simulink model "QP_NMPC_FSR"  (R2023a)
settings: Solver=ode4  StartTime=0.0  StopTime=T  RelTol=1e-3
InitFcn:
  | run('NLMPC_QUADCOPTER.m');
values from neighbouring files (symbols this model uses):
  g = 9.81    [NLMPC_QUADCOPTER.m]    (also in NMPC_XFcn.m)
  m = 0.85    [NLMPC_QUADCOPTER.m]    (also in NMPC_XFcn.m)
  PSI = zeros(1, length(PP))    [LOAD_NMPC.m]
undefined symbols (not defined in the file or in its folder): PP
libraries: robotcorelib x1, mpclib x1, uavutilslib x1
settings Model: ModifiedByFormat=salvatoregranata  Creator=salvatoregranata  LastModifiedBy=salvatoregranata

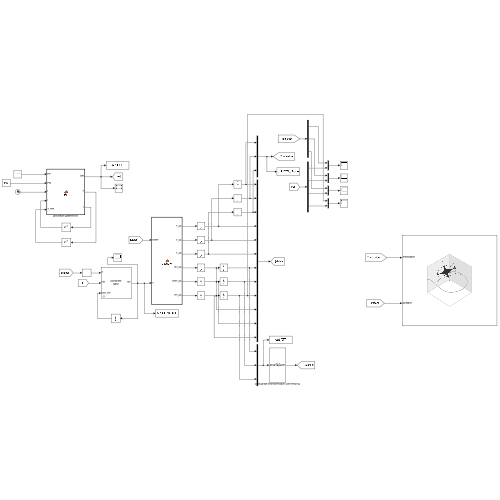
[thumbnail: Simulink's stored preview of the top-level diagram]
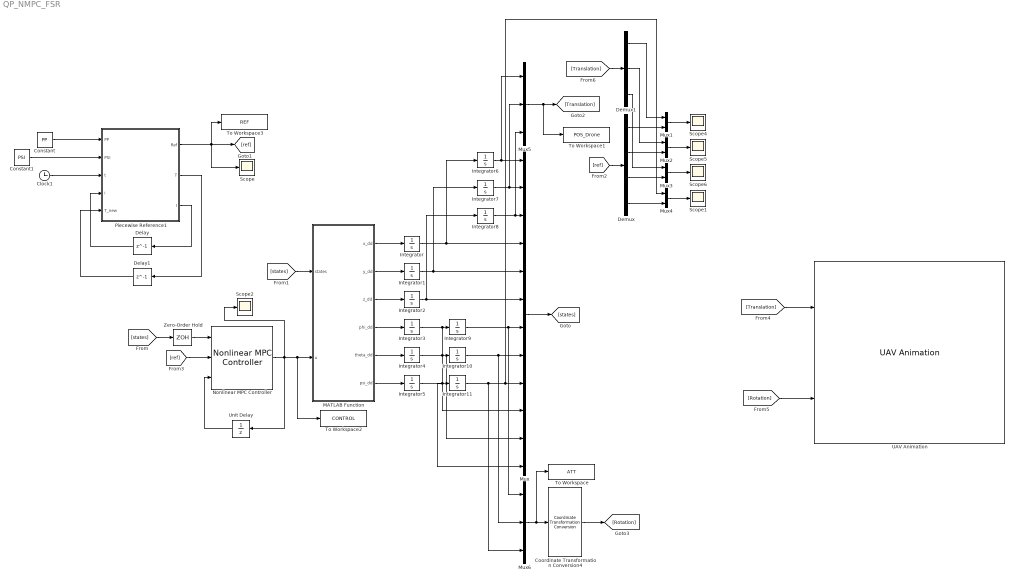
== system QP_NMPC_FSR ==
  Clock1 : Clock
  Constant : Constant  Value=PP
  Constant1 : Constant  Value=PSI
  Coordinate Transformation Conversion4 : robotcorelib/Coordinate Transformation Conversion  InputRepresentation=Euler Angles  InputEulerSequence=XYZ  ShowTrVecInputPort=on  OutputRepresentation=Quaternion  OutputEulerSequence=ZYX  ShowTrVecOutputPort=on  SimulateUsing=Interpreted execution
  Delay : Delay  DelayLength=1  InitialCondition=1  SampleTime=0.001
  Delay1 : Delay  DelayLength=1  SampleTime=0.001
  Demux : Demux
  Demux1 : Demux  Outputs=3
  Integrator{,1..5,9..10} (8 alike) : Integrator
  Integrator11 : Integrator  InitialCondition=PSI(1,1)
  Integrator6 : Integrator  InitialCondition=PP(1,1)
  Integrator7 : Integrator  InitialCondition=PP(2,1)
  Integrator8 : Integrator  InitialCondition=PP(3,1)
  MATLAB Function : MATLAB Function  TreatAsAtomicUnit=on
  Mux : Mux  Inputs=12
  Mux{1..4} (4 alike) : Mux  Inputs=2
  Mux5 : Mux  Inputs=3
  Mux6 : Mux  Inputs=3
  Nonlinear MPC Controller : mpclib/Nonlinear MPC Controller  nlmpcobj=my_NMPC  UseObjectTs=on  UseMEX=off  md_enabled=off  mvtarget_enabled=off  param_enabled=off  cost_enabled=off  mvseq_enabled=off  stateseq_enabled=off  ovseq_enabled=off  slack_enabled=off  status_enabled=off  ov_min=off  ov_max=off  mv_min=off  mv_max=off  mvrate_min=off  mvrate_max=off  state_min=off  state_max=off  ov_weight=off  mv_weight=off  mvrate_weight=off  ecr_weight=off  nlp_initialize=off
  Piecewise Reference1 : MATLAB Function  TreatAsAtomicUnit=on
  Scope{,1..2,4..6} (6 alike) : Scope
  To Workspace : ToWorkspace  VariableName=ATT  SaveFormat=Structure With Time  SampleTime=-1
  To Workspace1 : ToWorkspace  VariableName=POS_Drone  SaveFormat=Structure With Time  SampleTime=-1
  To Workspace2 : ToWorkspace  VariableName=CONTROL  SaveFormat=Structure With Time  SampleTime=-1
  To Workspace3 : ToWorkspace  VariableName=REF  SaveFormat=Structure With Time  SampleTime=-1
  UAV Animation : uavutilslib/UAV Animation  UAVType=Multirotor  UAVSize=1  InertialZDirection=Up  SampleTime=-1
  Unit Delay : UnitDelay  InitialCondition=m*g/4*ones(1,4)  SampleTime=-1  HasFrameUpgradeWarning=on
  Zero-Order Hold : ZeroOrderHold  SampleTime=0.01
  wires:
  Nonlinear MPC Controller/1 -> Unit Delay/1, Scope2/1, To Workspace2/1, MATLAB Function/2(u)
  Unit Delay/1 -> Nonlinear MPC Controller/3
  MATLAB Function/1(x_dd) -> Integrator/1
  MATLAB Function/2(y_dd) -> Integrator1/1
  MATLAB Function/3(z_dd) -> Integrator2/1
  MATLAB Function/4(phi_dd) -> Integrator3/1
  MATLAB Function/5(theta_dd) -> Integrator4/1
  MATLAB Function/6(psi_dd) -> Integrator5/1
  Integrator/1 -> Integrator6/1, Mux/4
  Integrator1/1 -> Integrator7/1, Mux/5
  Integrator2/1 -> Integrator8/1, Mux/6
  Integrator3/1 -> Mux/10, Integrator9/1
  Integrator4/1 -> Mux/11, Integrator10/1
  Integrator5/1 -> Mux/12, Integrator11/1
  Integrator6/1 -> Mux/1, Mux5/1
  Integrator9/1 -> Mux/7, Mux6/1
  Integrator10/1 -> Mux/8, Mux6/2
  Integrator11/1 -> Mux4/1, Mux/9, Mux6/3
  Mux/1 -> [states]
  [states] -> Zero-Order Hold/1
  Zero-Order Hold/1 -> Nonlinear MPC Controller/1
  [states] -> MATLAB Function/1(states)
  Clock1/1 -> Piecewise Reference1/3(t)
  Delay/1 -> Piecewise Reference1/4(i)
  Constant1/1 -> Piecewise Reference1/2(PSI)
  Piecewise Reference1/2(T) -> Delay1/1
  Delay1/1 -> Piecewise Reference1/5(T_new)
  Constant/1 -> Piecewise Reference1/1(PP)
  Piecewise Reference1/3(I) -> Delay/1
  [ref] -> Demux/1
  Demux/1 -> Mux1/2
  Mux1/1 -> Scope4/1
  Integrator7/1 -> Mux/2, Mux5/2
  Integrator8/1 -> Mux5/3, Mux/3
  Mux2/1 -> Scope5/1
  Demux/2 -> Mux2/2
  Mux3/1 -> Scope6/1
  Demux/3 -> Mux3/2
  [ref] -> Nonlinear MPC Controller/2
  Piecewise Reference1/1(Ref) -> To Workspace3/1, Scope/1, [ref]
  Mux5/1 -> To Workspace1/1, [Translation]
  [Translation] -> UAV Animation/1
  Mux6/1 -> To Workspace/1, Coordinate Transformation Conversion4/1
  Coordinate Transformation Conversion4/1 -> [Rotation]
  [Rotation] -> UAV Animation/2
  [Translation] -> Demux1/1
  Demux1/1 -> Mux1/1
  Demux1/2 -> Mux2/1
  Demux1/3 -> Mux3/1
  Demux/4 -> Mux4/2
  Mux4/1 -> Scope1/1

== matlab function QP_NMPC_FSR/MATLAB Function ==
  data: states input; u input; x_dd output size=1; y_dd output size=1; z_dd output size=1; phi_dd output size=1; theta_dd output size=1; psi_dd output size=1
function [x_dd,y_dd,z_dd,phi_dd,theta_dd,psi_dd] = QuadDyn(states,u)

% STATES
x=states(1);
y=states(2);
z=states(3);
x_d=states(4);
y_d=states(5);
z_d=states(6);
phi=states(7);
theta=states(8);
psi=states(9);
phi_d=states(10);
theta_d=states(11);
psi_d=states(12);

% INPUTS
u1=u(1);
u2=u(2);
u3=u(3);
u4=u(4);

% PARAMS
m=0.85;
d=2*0.15;
J=diag([2.5 2.1 4.3])*10^-3;
c=0.22;
g=9.81;

% DYNAMIC EQUATIONS
x_dd=sin(theta)/m*(u1+u2+u3+u4);
y_dd=-sin(phi)/m*(u1+u2+u3+u4);
z_dd=cos(phi)*cos(theta)/m*(u1+u2+u3+u4)-g;
phi_dd=d/J(1,1)*(u2-u4);
theta_dd=d/J(2,2)*(u1-u3);
psi_dd=c/J(3,3)*(-u1+u2-u3+u4);
end

== matlab function QP_NMPC_FSR/Piecewise Reference1 ==
  data: PP input; Ref output; PSI input; t input; i input; T_new input; T output; I output
function [Ref,T,I] = fcn(PP,PSI,t,i,T_new)
if t<=T_new+0.01

    I = i;
    T = T_new;
     
else

    I = i+1;
    T = T_new + 0.01;
    
end

Ref = [PP(1,I) PP(2,I) PP(3,I) PSI(I)];

end
